simulink model "biomasav_2"  (R2018a)
settings: Solver=ode8  StartTime=0.0  StopTime=10.0  FixedStep=0.0001  RelTol=1e-3
InitFcn:
  | SimulinkInit_linea_transmision
values from neighbouring files (symbols this model uses):
  b = 4.91    [SimulinkInit_linea_transmision.m]
  C = 1    [SimulinkInit_linea_transmision.m]
  C1 = 22e-6    (= 2.2e-05)    [SimulinkInit_linea_transmision.m]
  C2 = 22e-6    (= 2.2e-05)    [SimulinkInit_linea_transmision.m]
  C3 = 610e-6    (= 0.00061)    [SimulinkInit_linea_transmision.m]
  Cl = 20000e-6    (= 0.02)    [SimulinkInit_linea_transmision.m]
  Jd = 0.3    [SimulinkInit_linea_transmision.m]
  K = 25    [SimulinkInit_linea_transmision.m]    (also in uio_linear.m = K1+E*H)
  K1 = 9.66    [SimulinkInit_linea_transmision.m]    (also in uio_linear.m = K1')
  K11 = 0.8    [SimulinkInit_linea_transmision.m]
  K1d = 1.15    [SimulinkInit_linea_transmision.m]
  K2 = 6.97    [SimulinkInit_linea_transmision.m]
  K22 = 0.2    [SimulinkInit_linea_transmision.m]
  K2d = 1    [SimulinkInit_linea_transmision.m]
  K3 = 31.8    [SimulinkInit_linea_transmision.m]
  K33 = 0.23    [SimulinkInit_linea_transmision.m]
  K3d = 1    [SimulinkInit_linea_transmision.m]
  K4 = 15.1    [SimulinkInit_linea_transmision.m]
  Kd = 0.02    [SimulinkInit_linea_transmision.m]
  Kdc = 0.02    [SimulinkInit_linea_transmision.m]
  Kf = 1    [SimulinkInit_linea_transmision.m]
  Kh = 1.2    [SimulinkInit_linea_transmision.m]
  Ks = 21.5    [SimulinkInit_linea_transmision.m]
  Ksc = 3    [SimulinkInit_linea_transmision.m]
  Kv = 1    [SimulinkInit_linea_transmision.m]
  L = 5.2    [SimulinkInit_linea_transmision.m]
  L1 = 40e-3    (= 0.04)    [SimulinkInit_linea_transmision.m]
  L2 = 30e-3    (= 0.03)    [SimulinkInit_linea_transmision.m]
  L3 = 5e-3    (= 0.005)    [SimulinkInit_linea_transmision.m]
  L4 = 35e-6    (= 3.5e-05)    [SimulinkInit_linea_transmision.m]
  L5 = 22e-6    (= 2.2e-05)    [SimulinkInit_linea_transmision.m]
  L6 = 10e-6    (= 1e-05)    [SimulinkInit_linea_transmision.m]
  Pd = 0.1    [SimulinkInit_linea_transmision.m]
  R = 10    [SimulinkInit_linea_transmision.m]
  R1 = 0.1    [SimulinkInit_linea_transmision.m]
  R2 = 0.2    [SimulinkInit_linea_transmision.m]
  R3 = 1e-3    (= 0.001)    [SimulinkInit_linea_transmision.m]
  R4 = 0.005    [SimulinkInit_linea_transmision.m]
  R5 = 0.0012    [SimulinkInit_linea_transmision.m]
  R6 = 0.001    [SimulinkInit_linea_transmision.m]
  RL = 10    [SimulinkInit_linea_transmision.m]
  Sbin = 13.8    [SimulinkInit_linea_transmision.m]
  Svin = 2.91    [SimulinkInit_linea_transmision.m]
  T1 = 0.4    [SimulinkInit_linea_transmision.m]
  T2 = 1    [SimulinkInit_linea_transmision.m]
  T3 = 15    [SimulinkInit_linea_transmision.m]
  T4 = 2.5    [SimulinkInit_linea_transmision.m]
  T5 = 3.3    [SimulinkInit_linea_transmision.m]
  Tao1d = 0.5    [SimulinkInit_linea_transmision.m]
  Tao2d = 0.125    [SimulinkInit_linea_transmision.m]
  Tcd = 0.2    [SimulinkInit_linea_transmision.m]
  Tcr = 0.01    [SimulinkInit_linea_transmision.m]
  Tf = 0.04    [SimulinkInit_linea_transmision.m]
  Tr = 950    [SimulinkInit_linea_transmision.m]
  Tt = 450    [SimulinkInit_linea_transmision.m]
  Ttd = 0.04    [SimulinkInit_linea_transmision.m]
  Tv = 0.05    [SimulinkInit_linea_transmision.m]
  V = 20    [SimulinkInit_linea_transmision.m]
  wref = 70000    [SimulinkInit_linea_transmision.m]
  X_acid = 1.2    [SimulinkInit_linea_transmision.m]
  X_meth = 0.35    [SimulinkInit_linea_transmision.m]
  Z = 3    [SimulinkInit_linea_transmision.m]
libraries: dsparch4 x4, powerlib_meascontrol x2, simulink x1
settings Model: Creator=MarioAndres  LastModifiedBy=cmparedes
settings OptimizationCC: DefaultParameterBehavior=Inlined  EnhancedBackFolding=on  PassReuseOutputArgsAs=Individual arguments  OptimizeBlockOrder=speed  DifferentSizesBufferReuse=on  OptimizationCustomize=off
settings DebuggingCC: ParameterTunabilityLossMsg=error
settings HardwareCC: TargetBitPerPointer=64  TargetBitPerSizeT=64  TargetBitPerPtrDiffT=64  TargetLongLongMode=on  TargetIntDivRoundTo=Zero  TargetEndianess=LittleEndian  TargetWordSize=64  TargetHWDeviceType=MATLAB Host  ProdEqTarget=off
settings SFSimCC: MATLABDynamicMemAlloc=off
settings RTWCC: SystemTargetFile=ert.tlc  TemplateMakefile=ert_default_tmf  GenerateReport=on  IncludeHyperlinkInReport=on  LaunchReport=on  GenerateTraceInfo=on  GenerateTraceReport=on  GenerateTraceReportSl=on  GenerateTraceReportSf=on  GenerateTraceReportEml=on
settings CodeAppCC: ForceParamTrailComments=on  IgnoreCustomStorageClasses=off  OperatorAnnotations=on  SimulinkDataObjDesc=on  SFDataObjDesc=on  InsertBlockDesc=on
settings ERTTargetCC: TargetLangStandard=C99 (ISO)  GenerateSampleERTMain=on  SupportContinuousTime=on  InlinedParameterPlacement=NonHierarchical  ERTCustomFileTemplate=example_file_process.tlc

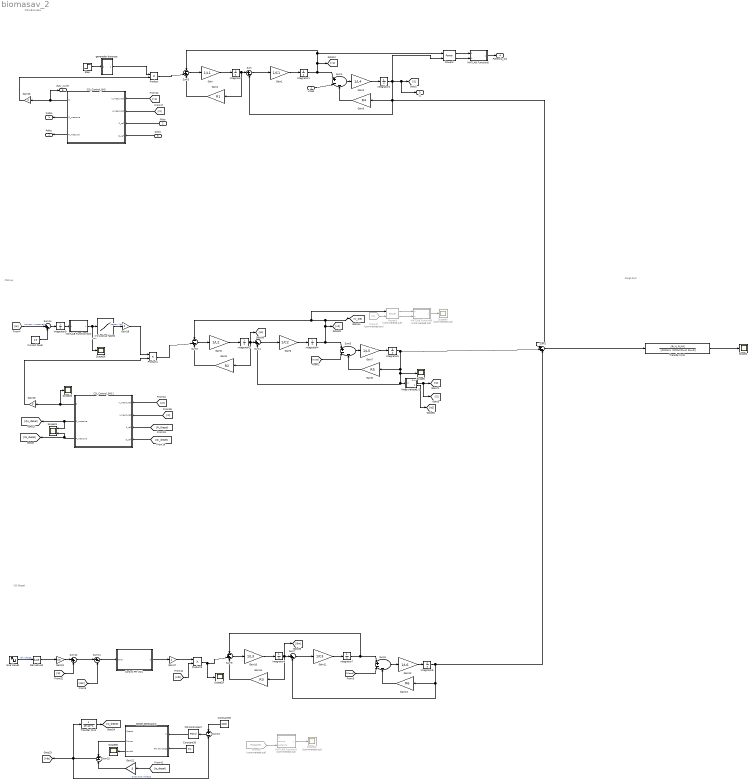
== system biomasav_2 ==
  note: CSI1-Biomasa
  note: CSI2-pv
  note: VSI-Diesel
  note: Carga RLC
  Vload : Inport
  Pibio : Inport  Port=2
  Qibio : Inport  Port=3
  1-D Lookup Table2 : Lookup_n-D  NumberOfTableDimensions=1  BreakpointsForDimension1=[0 10 20 30 40 50 70 80 100]  Table=[0 10 200 500 800 1000 1140 1150 1200]  InternalRulePriority=Speed  RndMeth=Simplest  InputSameDT=on
  CSI_Control_BIO : Subsystem  mask{A=[0.0201   -0.039932     0.01986], B=[1     -1.9966       0.998], T=0.0001, st_time=.1, Dn=[1     -1.0364], Dd=[1    -0.96364]}
      mask prompts: A "Numerador del control PR(z)"; B "Denominador del control PR(z)"; T "Tiempo de muestreo"; st_time "Tiempo_muerto"; Dn "Dn (Numerador de D(z))"; Dd "Dd (numerador de D(z))"
      mask DialogControl descripcion Prompt: Lazo de control de corriente para inversor monofasico. La entrada es un setpoint de potencia [P, Q]. Con ese setpoint se calcula la referencia de corriente sinusoidal deacuerdo a la tension medida de la red. Por lo anterior este controlador solo es valido para un inversor conectado a la red pues hara que se comporte como un CSI.
      mask DialogControl Control2 Prompt: Dn y Dd corresponden al numerador y denominador de la funcion de transferencia en Z (denominada D(z)) que hara un desfase de 90 de las señales medidas de tension y corriente del inversor. Estos desfases permiten mimificar las señales alfa y beta, de esta forma usar la misma teoria de potencia instantanea para el caso monofasico.
  CSI_Control_BIO1 : Subsystem  mask{A=[0.0201   -0.039932     0.01986], B=[1     -1.9966       0.998], T=0.0001, st_time=0, Dn=[1     -1.0364], Dd=[1    -0.96364]}
      mask prompts: A "Numerador del control PR(z)"; B "Denominador del control PR(z)"; T "Tiempo de muestreo"; st_time "Tiempo_muerto"; Dn "Dn (Numerador de D(z))"; Dd "Dd (numerador de D(z))"
      mask DialogControl descripcion Prompt: Lazo de control de corriente para inversor monofasico. La entrada es un setpoint de potencia [P, Q]. Con ese setpoint se calcula la referencia de corriente sinusoidal deacuerdo a la tension medida de la red. Por lo anterior este controlador solo es valido para un inversor conectado a la red pues hara que se comporte como un CSI.
      mask DialogControl Control2 Prompt: Dn y Dd corresponden al numerador y denominador de la funcion de transferencia en Z (denominada D(z)) que hara un desfase de 90 de las señales medidas de tension y corriente del inversor. Estos desfases permiten mimificar las señales alfa y beta, de esta forma usar la misma teoria de potencia instantanea para el caso monofasico.
  Constant29 : Constant  Value=1000
  Constant30 : Constant  Value=0.1
  Control PR VSI1 : Subsystem
  Current Panel : Constant  Value=1.5
  Derivative2 : Derivative  CoefficientInTFapproximation=0
  Diesel Generator2 : Subsystem
  From37 : From  Commented=on  GotoTag=Papadiel
  From47 : From  Commented=on  GotoTag=i2
  Gain : Gain  Gain=1/L1
  Gain1 : Gain  Gain=1/C1
  Gain10 : Gain  Gain=1/L3
  Gain11 : Gain  Gain=1/C3
  Gain12 : Gain  Gain=1/L6
  Gain13 : Gain  Gain=R6
  Gain14 : Gain  Gain=R3
  Gain{15..18} (4 alike) : Gain  Gain=2
  Gain19 : Gain  Gain=C3
  Gain2 : Gain  Gain=1/L4
  Gain21 : Gain  Gain=.5
  Gain3 : Gain  Gain=R4
  Gain4 : Gain  Gain=R1
  Gain5 : Gain  Gain=1/L2
  Gain6 : Gain  Gain=1/C2
  Gain7 : Gain  Gain=1/L5
  Gain8 : Gain  Gain=R5
  Gain9 : Gain  Gain=R2
  Integrator{,1..8} (9 alike) : Integrator
  Integrator9 : Integrator  LimitOutput=on  UpperSaturationLimit=1  LowerSaturationLimit=0
  "MATLAB Function SOC " : MATLAB Function  TreatAsAtomicUnit=on
  MATLAB Function3 : MATLAB Function  Commented=on  TreatAsAtomicUnit=on
  MATLAB Function5 : MATLAB Function  TreatAsAtomicUnit=on
  MATLAB Function6 : MATLAB Function  Commented=on  TreatAsAtomicUnit=on
  MeasureNode_I1 : Subsystem
  PID Controller2 : simulink/Continuous/PID Controller  Controller=PID  TimeDomain=Continuous-time  SampleTime=-1  IntegratorMethod=Forward Euler  FilterMethod=Forward Euler  Form=Parallel  UseFilter=on  ControllerParametersSource=internal  P=0.000853612192208084  I=3.94394231511782e-05  D=0.00224356290205903  N=0.155980576752107  InitialConditionSource=internal  InitialConditionForIntegrator=0  InitialConditionForFilter=0  ExternalReset=none  LimitOutput=off  UpperSaturationLimit=inf  LowerSaturationLimit=-inf  LinearizeAsGain=on  AntiWindupMode=none  Kb=1  TrackingMode=off  Kt=1  PParamMin=[]  PParamMax=[]  IParamMin=[]  IParamMax=[]  DParamMin=[]  DParamMax=[]  NParamMin=[]  NParamMax=[]  KbParamMin=[]  KbParamMax=[]  KtParamMin=[]  KtParamMax=[]  POutMin=[]  POutMax=[]  IOutMin=[]  IOutMax=[]  DOutMin=[]  DOutMax=[]  NOutMin=[]  NOutMax=[]  KbOutMin=[]  KbOutMax=[]  KtOutMin=[]  KtOutMax=[]  IntegratorOutMin=[]  IntegratorOutMax=[]  FilterOutMin=[]  FilterOutMax=[]  SumOutMin=[]  SumOutMax=[]  SumI1OutMin=[]  SumI1OutMax=[]  SumI2OutMin=[]  SumI2OutMax=[]  SumI3OutMin=[]  SumI3OutMax=[]  SumDOutMin=[]  SumDOutMax=[]  SaturationOutMin=[]  SaturationOutMax=[]  IntegratorContinuousStateAttributes=''  IntegratorStateMustResolveToSignalObject=off  IntegratorRTWStateStorageClass=Auto  FilterContinuousStateAttributes=''  FilterStateMustResolveToSignalObject=off  FilterRTWStateStorageClass=Auto  DifferentiatorICPrevScaledInput=0  DifferentiatorOutMin=[]  DifferentiatorOutMax=[]  InitialConditionSetting=State (most efficient)  FilterDiffOutCoefMin=[]  FilterDiffOutCoefMax=[]  SumDenOutMin=[]  SumDenOutMax=[]  SumNumOutMin=[]  SumNumOutMax=[]  ReciprocalOutMin=[]  ReciprocalOutMax=[]  DivideOutMin=[]  DivideOutMax=[]  TunerSelectOption=Transfer Function Based (PID Tuner App)
  Power3 : powerlib_meascontrol/Measurements/Power  Freq=60  Vinit=[1, 0]  Iinit=[1, 0]  Ts=0
      settings: SourceProductName=Simscape Power Systems
  Power4 : powerlib_meascontrol/Measurements/Power  Commented=on  Freq=60  Vinit=[1, 0]  Iinit=[1, 0]  Ts=0
      settings: SourceProductName=Simscape Power Systems
  Product : Product
  Product1 : Product
  Product3 : Product
  Scope{2,5,20,26,29,38} (6 alike) : Scope
  Scope21 : Scope  NumInputPorts=2
  Scope22 : Scope  Commented=on
  Scope40 : Scope  Commented=on
  Sine Wave1 : Sin  Amplitude=170  Frequency=2*pi*60  SampleTime=0
  Step : Step  Time=0  After=28  SampleTime=0
  Sum{,4,7,11} (4 alike) : Sum  Inputs=|+-
  Sum1 : Sum  Inputs=|+--
  Sum12 : Sum  Inputs=|++
  Sum13 : Sum  Inputs=+-
  Sum14 : Sum  Inputs=|++
  Sum15 : Sum  Inputs=+-
  Sum2 : Sum  Inputs=|+++
  Sum3 : Sum  Inputs=-|+-
  Sum5 : Sum  Inputs=|+--
  Sum6 : Sum  Inputs=-|+-
  Sum8 : Sum  Inputs=|+--
  Sum9 : Sum  Inputs=-|+-
  Transfer Fcn3 : TransferFcn  Numerator=[RL*L RL*R]  Denominator="[Cl*RL*L  (R*RL*Cl+L) RL+R]"
  Transfer Fcn4 : TransferFcn  Denominator=[1e-4 1]
  generador biomasa : Subsystem
  Qobio : Outport
  Pobio : Outport  Port=2
  i1 : Outport  Port=3
  Potencia_bio : Outport  Port=4
  duty_cycle : Outport  Port=5
  wires:
  MATLAB Function5/1(y) -> Potencia_bio/1
  CSI_Control_BIO/1(D) -> duty_cycle/1, Gain15/1
  Product/1 -> Sum3/2
  [i1] -> CSI_Control_BIO/2(I_measured)
  generador biomasa/1(Vdc) -> Product/1
  Step/1 -> generador biomasa/1(In1)
  Gain15/1 -> Product/2
  [v1] -> CSI_Control_BIO/1(V_measured)
  Sum/1 -> Gain1/1
  Sum3/1 -> Gain/1
  Gain4/1 -> Sum3/3
  Integrator1/1 -> [v1], Sum3/1, Power3/1, Sum1/1
  Gain2/1 -> Integrator2/1
  Sum1/1 -> Gain2/1
  Power3/1 -> MATLAB Function5/1(p)
  Gain1/1 -> Integrator1/1
  Power3/2 -> MATLAB Function5/2(q)
  Integrator/1 -> Gain4/1, Sum/1
  Gain/1 -> Integrator/1
  Gain3/1 -> Sum1/3
  Pibio/1 -> CSI_Control_BIO/3(P_ref)
  Qibio/1 -> CSI_Control_BIO/4(Q_ref)
  Vload/1 -> Sum1/2
  CSI_Control_BIO/2(Q_measure) -> Qobio/1
  CSI_Control_BIO/3(P_measure) -> Pobio/1
  [i2] -> CSI_Control_BIO1/2(I_measured)
  [Qi_diesel] -> CSI_Control_BIO1/4(Q_ref)
  Gain16/1 -> Product1/2
  Sum6/1 -> Gain5/1
  [i3] -> Sum12/2
  Gain11/1 -> Integrator7/1
  MeasureNode_I1/2(Out1) -> [a2]
  MATLAB Function3/1(y) -> Scope22/1
  Current Panel/1 -> Sum14/2
  MATLAB Function6/1(y) -> Scope40/1
  Gain17/1 -> Product3/1
  CSI_Control_BIO1/1(D) -> Scope20/1, Gain16/1
  Sum8/1 -> Gain12/1
  PID Controller2/1 -> Diesel Generator2/1(in)
  [i3m] -> Sum11/2
  Sum15/1 -> [Vdc], Sum13/2, Transfer Fcn4/1  "Output DC Voltage"
  [Vload] -> Sum8/2
  "MATLAB Function SOC "/1(y) -> Scope26/1, 1-D Lookup Table2/1  "soc"
  Diesel Generator2/2(Power) -> Sum15/1
  Sum9/1 -> Gain10/1
  Gain5/1 -> Integrator3/1
  [v2] -> CSI_Control_BIO1/1(V_measured)
  Gain6/1 -> Integrator4/1
  Power4/1 -> MATLAB Function6/1(p)
  [Pi_Diesel] -> CSI_Control_BIO1/3(P_ref)
  Power4/2 -> MATLAB Function6/2(q)
  Constant29/1 -> Sum13/1
  Gain21/1 -> Sum15/2
  [Vdc] -> Product3/2
  Diesel Generator2/3(caudal) -> Scope38/1
  Transfer Fcn4/1 -> [Io_diesel]
  Constant30/1 -> Diesel Generator2/2(Par de Carga)
  From37/1 -> MATLAB Function3/3(potencia)
  Sum13/1 -> PID Controller2/1
  Integrator4/1 -> [v2], [V_die], Power4/1, Sum6/1, Sum5/1
  Sum14/1 -> Integrator9/1
  Gain18/1 -> Product1/1
  Sum11/1 -> Control PR VSI1/1(Ierror)
  Gain13/1 -> Sum8/3
  Derivative2/1 -> Gain19/1
  1-D Lookup Table2/1 -> Gain18/1  "battery Vdc"
  Integrator9/1 -> "MATLAB Function SOC "/1(u)
  Product1/1 -> Sum6/2
  From47/1 -> Power4/2
  Sum4/1 -> Gain6/1
  Control PR VSI1/1(d) -> Gain17/1
  Product3/1 -> Sum9/2, Scope29/1
  Integrator7/1 -> Sum9/1, Sum8/1
  Integrator5/1 -> Sum2/2, Scope5/1, MeasureNode_I1/1(in), Sum4/2, Gain8/1
  Gain7/1 -> Integrator5/1
  [Io_diesel] -> Gain21/1
  [Vload] -> Sum5/2
  CSI_Control_BIO1/3(P_measure) -> [Po_diesel], Scope21/2
  Gain12/1 -> Integrator8/1
  CSI_Control_BIO1/2(Q_measure) -> [Qo_diesel], Scope21/1
  Transfer Fcn3/1 -> Scope2/1
  Gain8/1 -> Sum5/3
  Sine Wave1/1 -> Derivative2/1  "ref voltage"
  Gain9/1 -> Sum6/3
  [ipi] -> Sum14/1  "inductor I measured"
  Gain10/1 -> Integrator6/1
  Integrator2/1 -> Power3/2, Sum2/1, Sum/2, Gain3/1, i1/1, [i1]
  Gain19/1 -> Sum12/1
  Sum5/1 -> Gain7/1
  Gain14/1 -> Sum9/3
  Sum2/1 -> Transfer Fcn3/1
  Integrator8/1 -> Sum2/3, Gain13/1, Sum7/2
  Sum12/1 -> Sum11/1
  Integrator6/1 -> [i3m], Gain14/1, Sum7/1
  MeasureNode_I1/1(Out) -> [i2], [I2]
  Integrator3/1 -> [ipi], Gain9/1, Sum4/1
  Sum7/1 -> Gain11/1

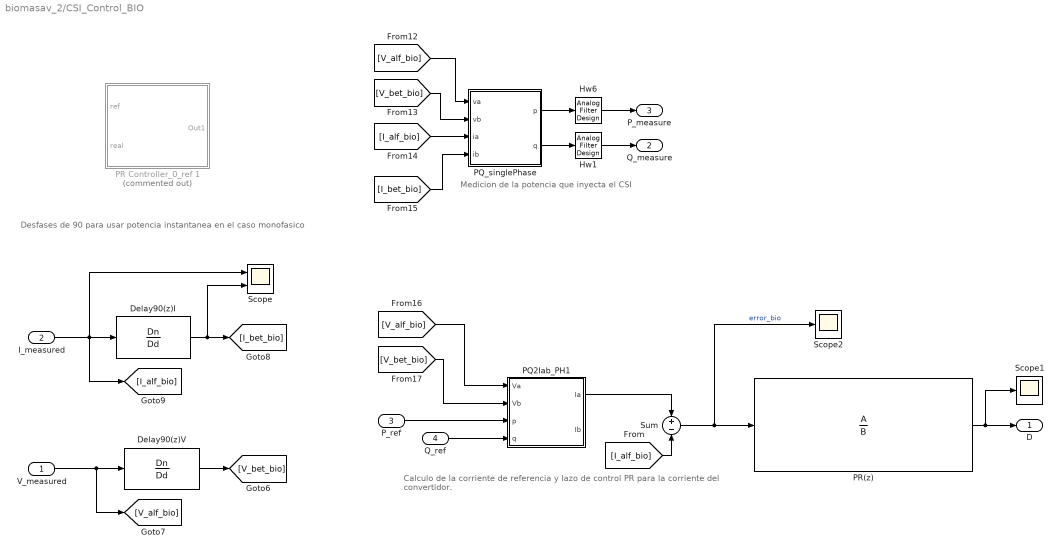
== system biomasav_2/CSI_Control_BIO ==
  note: Medicion de la potencia que inyecta el CSI
  note: Desfases de 90 para usar potencia
      | instantanea en el caso monofasico
  note: Calculo de la corriente de referencia
      | y lazo de control PR para la corriente
      | del convertidor.
  V_measured : Inport
  I_measured : Inport  Port=2
  P_ref : Inport  Port=3
  Q_ref : Inport  Port=4
  Delay90(z)I : DiscreteTransferFcn  Numerator=Dn  Denominator=Dd  SampleTime=T
  Delay90(z)V : DiscreteTransferFcn  Numerator=Dn  Denominator=Dd  SampleTime=T
  Hw1 : dsparch4/Analog Filter Design  method=Bessel  filttype=Lowpass  N=4  Wlo=30*2*pi  Whi=80  Rp=2  Rs=80
  Hw6 : dsparch4/Analog Filter Design  method=Bessel  filttype=Lowpass  N=4  Wlo=30*2*pi  Whi=80  Rp=2  Rs=80
  PQ2Iab_PH1 : MATLAB Function  TreatAsAtomicUnit=on
  PQ_singlePhase : MATLAB Function  TreatAsAtomicUnit=on
  PR Controller_0_ref 1 : Subsystem  Commented=on  mask{Kp=40/100, Ki=200, wa=2, w0=60*2*pi, st_time=1e-3}
      mask prompts: Kp "Ganancia Proporcional"; Ki "Ganancia Integral"; wa "Ancho camapana resonancia"; w0 "Frecuencia Central"; st_time "Tiempo muerto (Start)"
      mask Display:
      | port_label('input',1,'ref')
      | port_label('input',2,'sens')
      | port_label('output',1,'out')
      | 
      | plot(.4+[0:.01:pi/10], .32+sin(40*[0:.01:pi/10])/13)
      | 
      | plot([.4 .6],.05+[.5 .7])
      | plot([.4 .6],.05+[.9 .7])
      | plot([.4 .4],.05+[.9 .5])
      | 
      | text(.27,.37,'\fontsize{25} \int', 'texmode', 'on')
  PR(z) : DiscreteTransferFcn  Numerator=A  Denominator=B  SampleTime=T
  Scope : Scope  NumInputPorts=2
  Scope1 : Scope
  Scope2 : Scope
  Sum : Sum  Inputs=+-
  D : Outport
  Q_measure : Outport  Port=2
  P_measure : Outport  Port=3
  wires:
  I_measured/1 -> Scope/1, Delay90(z)I/1, [I_alf_bio]
  [V_bet_bio] -> PQ2Iab_PH1/2(Vb)
  Delay90(z)I/1 -> Scope/2, [I_bet_bio]
  [I_bet_bio] -> PQ_singlePhase/4(ib)
  [I_alf_bio] -> PQ_singlePhase/3(ia)
  [V_alf_bio] -> PQ2Iab_PH1/1(Va)
  Delay90(z)V/1 -> [V_bet_bio]
  [V_bet_bio] -> PQ_singlePhase/2(vb)
  [V_alf_bio] -> PQ_singlePhase/1(va)
  V_measured/1 -> Delay90(z)V/1, [V_alf_bio]
  P_ref/1 -> PQ2Iab_PH1/3(p)
  Q_ref/1 -> PQ2Iab_PH1/4(q)
  Sum/1 -> Scope2/1, PR(z)/1  "error_bio"
  [I_alf_bio] -> Sum/2
  PQ2Iab_PH1/1(Ia) -> Sum/1
  PR(z)/1 -> Scope1/1, D/1
  PQ_singlePhase/2(q) -> Hw1/1
  Hw1/1 -> Q_measure/1
  PQ_singlePhase/1(p) -> Hw6/1
  Hw6/1 -> P_measure/1

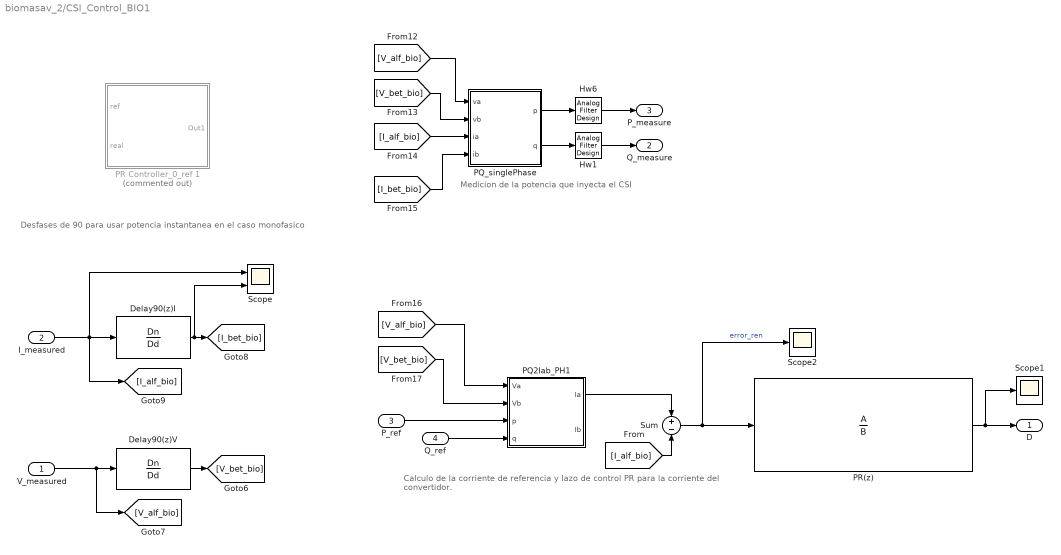
== system biomasav_2/CSI_Control_BIO1 ==
  note: Medicion de la potencia que inyecta el CSI
  note: Desfases de 90 para usar potencia
      | instantanea en el caso monofasico
  note: Calculo de la corriente de referencia
      | y lazo de control PR para la corriente
      | del convertidor.
  V_measured : Inport
  I_measured : Inport  Port=2
  P_ref : Inport  Port=3
  Q_ref : Inport  Port=4
  Delay90(z)I : DiscreteTransferFcn  Numerator=Dn  Denominator=Dd  SampleTime=T
  Delay90(z)V : DiscreteTransferFcn  Numerator=Dn  Denominator=Dd  SampleTime=T
  Hw1 : dsparch4/Analog Filter Design  method=Bessel  filttype=Lowpass  N=4  Wlo=30*2*pi  Whi=80  Rp=2  Rs=80
  Hw6 : dsparch4/Analog Filter Design  method=Bessel  filttype=Lowpass  N=4  Wlo=30*2*pi  Whi=80  Rp=2  Rs=80
  PQ2Iab_PH1 : MATLAB Function  TreatAsAtomicUnit=on
  PQ_singlePhase : MATLAB Function  TreatAsAtomicUnit=on
  PR Controller_0_ref 1 : Subsystem  Commented=on  mask{Kp=40/100, Ki=200, wa=2, w0=60*2*pi, st_time=1e-3}
      mask prompts: Kp "Ganancia Proporcional"; Ki "Ganancia Integral"; wa "Ancho camapana resonancia"; w0 "Frecuencia Central"; st_time "Tiempo muerto (Start)"
      mask Display:
      | port_label('input',1,'ref')
      | port_label('input',2,'sens')
      | port_label('output',1,'out')
      | 
      | plot(.4+[0:.01:pi/10], .32+sin(40*[0:.01:pi/10])/13)
      | 
      | plot([.4 .6],.05+[.5 .7])
      | plot([.4 .6],.05+[.9 .7])
      | plot([.4 .4],.05+[.9 .5])
      | 
      | text(.27,.37,'\fontsize{25} \int', 'texmode', 'on')
  PR(z) : DiscreteTransferFcn  Numerator=A  Denominator=B  SampleTime=T
  Scope : Scope  NumInputPorts=2
  Scope1 : Scope
  Scope2 : Scope
  Sum : Sum  Inputs=+-
  D : Outport
  Q_measure : Outport  Port=2
  P_measure : Outport  Port=3
  wires:
  I_measured/1 -> Scope/1, Delay90(z)I/1, [I_alf_bio]
  [V_bet_bio] -> PQ2Iab_PH1/2(Vb)
  Delay90(z)I/1 -> Scope/2, [I_bet_bio]
  [I_bet_bio] -> PQ_singlePhase/4(ib)
  [I_alf_bio] -> PQ_singlePhase/3(ia)
  [V_alf_bio] -> PQ2Iab_PH1/1(Va)
  Delay90(z)V/1 -> [V_bet_bio]
  [V_bet_bio] -> PQ_singlePhase/2(vb)
  [V_alf_bio] -> PQ_singlePhase/1(va)
  V_measured/1 -> Delay90(z)V/1, [V_alf_bio]
  P_ref/1 -> PQ2Iab_PH1/3(p)
  Q_ref/1 -> PQ2Iab_PH1/4(q)
  Sum/1 -> Scope2/1, PR(z)/1  "error_ren"
  [I_alf_bio] -> Sum/2
  PQ2Iab_PH1/1(Ia) -> Sum/1
  PR(z)/1 -> Scope1/1, D/1
  PQ_singlePhase/2(q) -> Hw1/1
  Hw1/1 -> Q_measure/1
  PQ_singlePhase/1(p) -> Hw6/1
  Hw6/1 -> P_measure/1

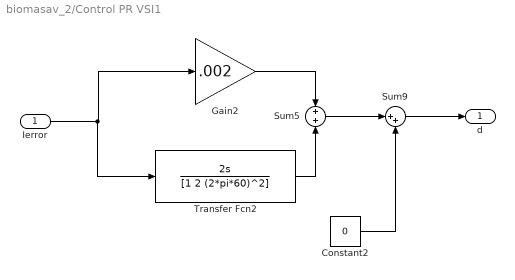
== system biomasav_2/Control PR VSI1 ==
  Ierror : Inport
  Constant2 : Constant  Value=0
  Gain2 : Gain  Gain=.002
  Sum5 : Sum  Inputs=+|+
  Sum9 : Sum  Inputs=|++
  Transfer Fcn2 : TransferFcn  Numerator=[2 0]  Denominator=[1 2 (2*pi*60)^2]
  d : Outport
  wires:
  Constant2/1 -> Sum9/2
  Sum5/1 -> Sum9/1
  Transfer Fcn2/1 -> Sum5/2
  Gain2/1 -> Sum5/1
  Ierror/1 -> Transfer Fcn2/1, Gain2/1
  Sum9/1 -> d/1

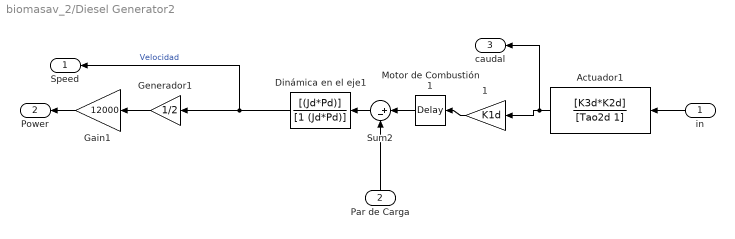
== system biomasav_2/Diesel Generator2 ==
  in : Inport
  Par de Carga : Inport  Port=2
  " 1" : Gain  Gain=K1d
  " Generador1" : Gain  Gain=1/2
  Actuador1 : TransferFcn  Numerator=[K3d*K2d]  Denominator=[Tao2d 1]
  Dinámica en el eje1 : TransferFcn  Numerator=[(Jd*Pd)]  Denominator=[1 (Jd*Pd)]
  Gain1 : Gain  Gain=12000
  Motor de Combustión1 : TransportDelay  DelayTime=Tao1d
  Sum2 : Sum  Inputs=|+-
  Speed : Outport
  Power : Outport  Port=2
  caudal : Outport  Port=3
  wires:
  " 1"/1 -> Motor de Combustión1/1
  " Generador1"/1 -> Gain1/1
  Motor de Combustión1/1 -> Sum2/1
  Actuador1/1 -> caudal/1, " 1"/1
  Dinámica en el eje1/1 -> Speed/1, " Generador1"/1  "Velocidad"
  Sum2/1 -> Dinámica en el eje1/1
  in/1 -> Actuador1/1
  Par de Carga/1 -> Sum2/2
  Gain1/1 -> Power/1

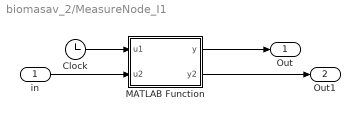
== system biomasav_2/MeasureNode_I1 ==
  in : Inport
  Clock : Clock
  MATLAB Function : MATLAB Function  TreatAsAtomicUnit=on
  Out : Outport
  Out1 : Outport  Port=2
  wires:
  MATLAB Function/1(y) -> Out/1
  Clock/1 -> MATLAB Function/1(u1)
  in/1 -> MATLAB Function/2(u2)
  MATLAB Function/2(y2) -> Out1/1

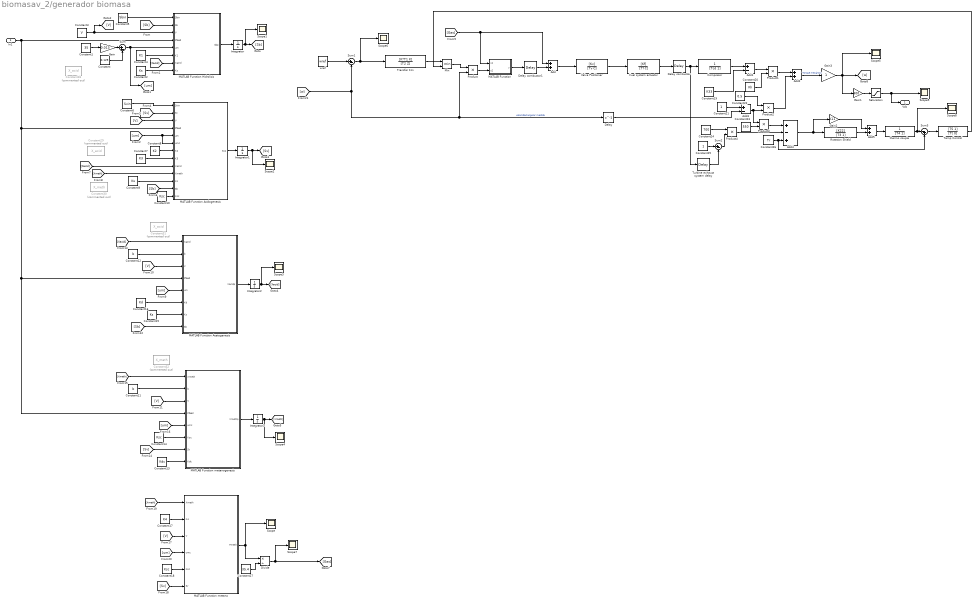
== system biomasav_2/generador biomasa ==
  In1 : Inport
  Add : Sum
  Add1 : Sum  Inputs=+-
  Add2 : Sum
  Add3 : Sum  Inputs=+-
  Add4 : Sum  Inputs=+-+
  Add5 : Sum
  Compresor : TransferFcn  Denominator=[Tcd 1]
  Constant : Constant  Value=0.129
  Constant1 : Constant  Value=35
  Constant10 : Constant  Value=Ksc
  Constant11 : Constant  Value=b
  Constant12 : Constant  Value=b
  Constant13 : Constant  Value=Kdc
  Constant14 : Constant  Value=Ksc
  Constant15 : Constant  Value=Ks
  Constant16 : Constant  Value=Kd
  Constant17 : Constant  Value=K4
  Constant18 : Constant  Value=Ksc
  Constant19 : Constant  Value=K33
  Constant2 : Constant  Value=Ks
  Constant20 : Constant  Value=Kh
  Constant21 : Constant
  Constant22 : Constant  Value=0.5
  Constant23 : Constant  Value=550
  Constant24 : Constant  Value=700
  Constant25 : Constant
  Constant26 : Constant  Value=Tr
  Constant27 : Constant  Value=35.4
  Constant28 : Constant  Commented=on  Value=X_acid
  Constant29 : Constant  Commented=on  Value=X_acid
  Constant3 : Constant  Value=V
  Constant30 : Constant  Commented=on  Value=X_meth
  Constant31 : Constant  Commented=on  Value=X_acid
  Constant32 : Constant  Commented=on  Value=X_meth
  Constant4 : Constant  Value=K1
  Constant5 : Constant  Value=Sbin
  Constant6 : Constant  Value=Svin
  Constant7 : Constant  Value=K3
  Constant8 : Constant  Value=K2
  Constant9 : Constant  Value=Ks
  Delay : Delay  DelayLength=1
  Delay combustor : TransportDelay  DelayTime=Tcr
  Delay combustor1 : TransportDelay  DelayTime=0
  Divide : Product  Inputs=*/
  Fuel system actuator : TransferFcn  Numerator=[Kf]  Denominator=[Tf C]
  Gain : Gain  Gain=0.013
  Gain1 : Gain  Gain=900
  Gain2 : Gain  Gain=K11
  Gain3 : Gain
  Integrator : Integrator
  Integrator1 : Integrator
  Integrator2 : Integrator  InitialCondition=1.2
  Integrator3 : Integrator  InitialCondition=0.35
  MATLAB Function : MATLAB Function  TreatAsAtomicUnit=on
  MATLAB Function Acetogenesis : MATLAB Function  TreatAsAtomicUnit=on
  MATLAB Function Acidogenesis : MATLAB Function  TreatAsAtomicUnit=on
  MATLAB Function Hidrolisis : MATLAB Function  TreatAsAtomicUnit=on
  MATLAB Function metano : MATLAB Function  TreatAsAtomicUnit=on
  MATLAB Function metanogenesis : MATLAB Function  TreatAsAtomicUnit=on
  Min : MinMax  Inputs=2
  Product{,1..4} (5 alike) : Product
  Rotation Shield : TransferFcn  Numerator=[K22]  Denominator=[T3 1]
  Saturation : Saturate  UpperLimit=1000  LowerLimit=0
  Scope{,1..9} (10 alike) : Scope
  Sum : Sum  Inputs=|+-
  Sum1 : Sum  Inputs=|+-
  Sum2 : Sum  Inputs=|+-
  Sum3 : Sum  Inputs=|-+
  Temp Control : TransferFcn  Numerator=[T5 1]  Denominator=[Tt 0]
  Transfer Fcn : TransferFcn  Numerator=[K*T1 K]  Denominator=[T2 Z]
  Turbine exhaust system delay : TransportDelay  DelayTime=Ttd
  Valve Positioner : TransferFcn  Numerator=[Kv]  Denominator=[Tv C]
  thermo couple : TransferFcn  Denominator=[T4 1]
  wref : Constant  Value=wref
  Vdc : Outport
  wires:
  MATLAB Function metano/1(Fmeth) -> Divide/1, Scope/1
  Sum/1 -> [um], MATLAB Function Hidrolisis/5(um)
  Constant16/1 -> MATLAB Function Acetogenesis/6(Kd)
  Temp Control/1 -> Min/2
  Integrator/1 -> Scope1/1, [Sb]
  Gain3/1 -> Gain1/1, Scope5/1, [w]
  Sum1/1 -> Transfer Fcn/1, Scope6/1
  [Sb] -> MATLAB Function Acetogenesis/8(Sb)
  [Sv] -> MATLAB Function metanogenesis/7(Sv)
  Add4/1 -> Rotation Shield/1, Gain2/1
  Constant8/1 -> MATLAB Function Acidogenesis/7(K2)
  Constant24/1 -> Product4/1
  [V] -> MATLAB Function Acetogenesis/3(V)
  Constant23/1 -> Product3/2
  Constant27/1 -> Divide/2
  [Sb] -> MATLAB Function Acidogenesis/12(Sb)
  Integrator3/1 -> Scope4/1, [Xmeth]
  Integrator2/1 -> Scope3/1, [Xacid]
  Divide/1 -> Scope7/1, [Gas]
  Constant7/1 -> MATLAB Function Acidogenesis/8(K3)
  Delay combustor/1 -> Turbine exhaust system delay/1, Compresor/1
  [V] -> MATLAB Function Acidogenesis/3(V)
  Constant12/1 -> MATLAB Function Acetogenesis/2(b)
  Sum2/1 -> Product4/2
  [V] -> MATLAB Function metanogenesis/3(V)
  Gain/1 -> Sum/1
  Product/1 -> MATLAB Function/2(u2)
  [w] -> Product/2, Delay/1, Sum1/2  "velocidad angular medida"
  Constant6/1 -> MATLAB Function Acidogenesis/1(Svin)
  wref/1 -> Sum1/1
  [Gas] -> MATLAB Function/1(u1), Add/1
  [Sv] -> MATLAB Function metano/6(Sv)
  MATLAB Function Hidrolisis/1(Sbp) -> Integrator/1
  Turbine exhaust system delay/1 -> Sum2/2
  MATLAB Function Acetogenesis/1(Xacidp) -> Integrator2/1
  Constant/1 -> Sum/2
  Constant18/1 -> MATLAB Function metano/5(Ksc)
  In1/1 -> MATLAB Function Acidogenesis/4(Ffeed), MATLAB Function metanogenesis/4(Ffeed), MATLAB Function Acetogenesis/4(Ffeed), MATLAB Function Hidrolisis/4(Ffeed)
  Add3/1 -> Product3/1, Product2/2
  [um] -> MATLAB Function Acetogenesis/5(um)
  Product3/1 -> Add4/1
  Constant15/1 -> MATLAB Function Acetogenesis/7(Ks)
  thermo couple/1 -> Scope8/1, Sum3/1
  Fuel system actuator/1 -> Delay combustor/1
  Add/1 -> Valve Positioner/1
  Add5/1 -> thermo couple/1
  Gain2/1 -> Add5/1
  Constant22/1 -> Product2/1
  [um] -> MATLAB Function metano/4(umc)
  Compresor/1 -> Add1/1
  Constant10/1 -> MATLAB Function Acidogenesis/13(Ksc)
  [um] -> MATLAB Function Acidogenesis/6(umc), MATLAB Function Acidogenesis/5(um)
  Constant9/1 -> MATLAB Function Acidogenesis/11(Ks)
  Constant1/1 -> Gain/1
  Constant13/1 -> MATLAB Function metanogenesis/8(Kdc)
  Constant26/1 -> Sum3/2, Add4/3
  Integrator1/1 -> Scope2/1, [Sv]
  [Xmeth] -> MATLAB Function metanogenesis/1(Xmeth)
  Add2/1 -> Gain3/1  "Torque mecánico"
  MATLAB Function/1(y) -> Delay combustor1/1
  Saturation/1 -> Vdc/1, Scope9/1
  [Sb] -> MATLAB Function Hidrolisis/2(Sb)
  Min/1 -> Product/1
  Constant3/1 -> [V], MATLAB Function Hidrolisis/3(V)
  MATLAB Function Acidogenesis/1(Svp) -> Integrator1/1
  Constant5/1 -> MATLAB Function Hidrolisis/1(Sbin)
  Constant20/1 -> Product1/2
  [Xmeth] -> MATLAB Function Acidogenesis/10(Xmeth)
  Sum3/1 -> Temp Control/1
  Gain1/1 -> Saturation/1
  Constant21/1 -> Add3/1
  Constant25/1 -> Sum2/1
  Product2/1 -> Add2/2
  [Xacid] -> MATLAB Function Acidogenesis/9(Xacid)
  Valve Positioner/1 -> Fuel system actuator/1
  Constant4/1 -> MATLAB Function Hidrolisis/6(K1)
  Constant11/1 -> MATLAB Function metanogenesis/2(b)
  Rotation Shield/1 -> Add5/2
  Add1/1 -> Product1/1
  [Sv] -> MATLAB Function Acidogenesis/2(Sv)
  [Xacid] -> MATLAB Function Acetogenesis/1(Xacid)
  Constant19/1 -> Add1/2
  Product1/1 -> Add2/1
  Transfer Fcn/1 -> Min/1
  Delay combustor1/1 -> Add/2
  [um] -> MATLAB Function metanogenesis/5(umc)
  MATLAB Function metanogenesis/1(Xmethp) -> Integrator3/1
  Constant14/1 -> MATLAB Function metanogenesis/6(Ksc)
  Product4/1 -> Add4/2
  Constant2/1 -> MATLAB Function Hidrolisis/8(Ks)
  Constant17/1 -> MATLAB Function metano/2(K4)
  [V] -> MATLAB Function metano/3(V)
  [Xmeth] -> MATLAB Function metano/1(Xmeth)
  [Xacid] -> MATLAB Function Hidrolisis/7(Xacid)
  Delay/1 -> Add3/2

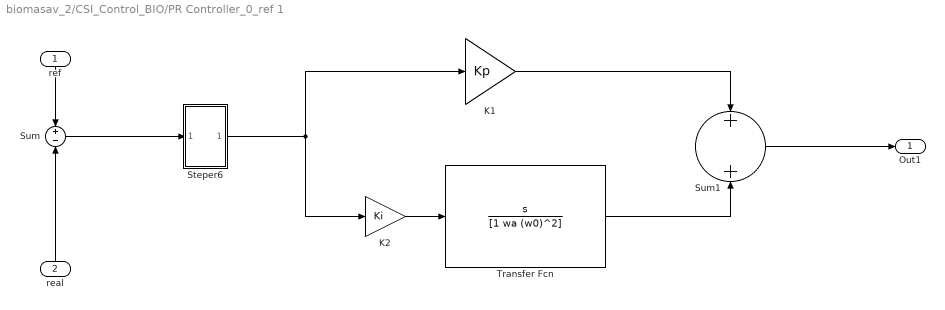
== system biomasav_2/CSI_Control_BIO/PR Controller_0_ref 1 ==
  ref : Inport
  real : Inport  Port=2
  K1 : Gain  Gain=Kp
  K2 : Gain  Gain=Ki
  Steper6 : Subsystem
  Sum : Sum  Inputs=+-
  Sum1 : Sum  Inputs=+|+
  Transfer Fcn : TransferFcn  Numerator=[1 0]  Denominator=[1 wa (w0)^2]
  Out1 : Outport
  wires:
  real/1 -> Sum/2
  ref/1 -> Sum/1
  Sum/1 -> Steper6/1(In1)
  K1/1 -> Sum1/1
  Transfer Fcn/1 -> Sum1/2
  K2/1 -> Transfer Fcn/1
  Steper6/1(Out1) -> K1/1, K2/1
  Sum1/1 -> Out1/1

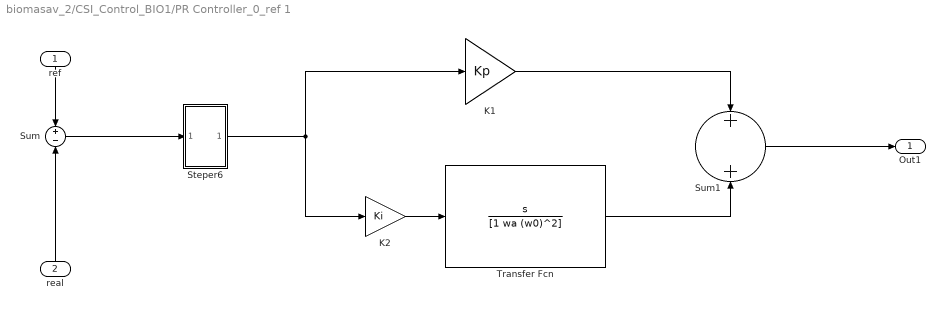
== system biomasav_2/CSI_Control_BIO1/PR Controller_0_ref 1 ==
  ref : Inport
  real : Inport  Port=2
  K1 : Gain  Gain=Kp
  K2 : Gain  Gain=Ki
  Steper6 : Subsystem
  Sum : Sum  Inputs=+-
  Sum1 : Sum  Inputs=+|+
  Transfer Fcn : TransferFcn  Numerator=[1 0]  Denominator=[1 wa (w0)^2]
  Out1 : Outport
  wires:
  real/1 -> Sum/2
  ref/1 -> Sum/1
  Sum/1 -> Steper6/1(In1)
  K1/1 -> Sum1/1
  Transfer Fcn/1 -> Sum1/2
  K2/1 -> Transfer Fcn/1
  Steper6/1(Out1) -> K1/1, K2/1
  Sum1/1 -> Out1/1

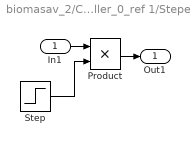
== system biomasav_2/CSI_Control_BIO/PR Controller_0_ref 1/Steper6 ==
  In1 : Inport
  Product : Product
  Step : Step  Time=st_time  SampleTime=0
  Out1 : Outport
  wires:
  Product/1 -> Out1/1
  In1/1 -> Product/1
  Step/1 -> Product/2

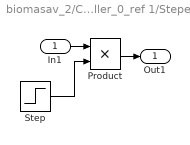
== system biomasav_2/CSI_Control_BIO1/PR Controller_0_ref 1/Steper6 ==
  In1 : Inport
  Product : Product
  Step : Step  Time=st_time  SampleTime=0
  Out1 : Outport
  wires:
  Product/1 -> Out1/1
  In1/1 -> Product/1
  Step/1 -> Product/2

== matlab function biomasav_2/CSI_Control_BIO/PQ_singlePhase ==
  data: va input; p output; vb input; ia input; ib input; q output
function [p, q] = fcn(va, vb, ia, ib)
% Esta funcion calcula la potencia activa y reactiva instantanea
% para el caso mnosofasico. En la revision de 2 papers he observado
% que una manera de extender la teoria de potencia al caso monofasico
% es asumiendo la tension o corriente de una fase como la componente
% alpha y hacer un desfase de 90 grados para obtener una version
% artificial de beta.

paux=va*ia+vb*ib;
if(paux > 20e4)
    paux = 20e4;
end
if(paux < -20e4)
    paux = -20e-4;
end

p = paux/2; % potencia activa instantanea

qaux = vb*ia-va*ib;

if(qaux>20e4)
    qaux=20e4;
end
if(qaux<-20e4)
    qaux=-20e4;
end

q = qaux/2; % potencia reactiva instantanea

== matlab function biomasav_2/CSI_Control_BIO1/PQ2Iab_PH1 ==
  data: Va input; Ia output; Vb input; p input; q input; Ib output
function [Ia, Ib] = fcn(Va, Vb, p, q)
%#codegen
% Ia=0;
% Ib=0;
% divide by zero protection
if(abs((Va^2+Vb^2))<=1000*eps(0))
    det = 1/eps(0);
else
    det = 1/(Va^2+Vb^2); % constante auxiliar
end
%det = 1/(Va^2+Vb^2);

Mat = det*[Va Vb; Vb -Va];

Iab = Mat*[2*p;2*q];

Iaaux = Iab(1);
Ibaux = Iab(2);

ilim=1e3;

if(Iaaux>ilim)
    Iaaux=ilim;
end
if(Iaaux<-ilim)
    Iaaux =-ilim;    
end

if(isnan(Iaaux))
    Iaaux=0;
end
%-----------------


if(Ibaux>ilim)
    Ibaux=ilim;
end
if(Ibaux<-ilim)
    Ibaux =-ilim;    
end

if(isnan(Ibaux))
    Ibaux=0;
end
%-----------------


Ia = Iaaux;
Ib = Ibaux;

== matlab function biomasav_2/CSI_Control_BIO1/PQ_singlePhase ==
  data: va input; p output; vb input; ia input; ib input; q output
function [p, q] = fcn(va, vb, ia, ib)
% Esta funcion calcula la potencia activa y reactiva instantanea
% para el caso mnosofasico. En la revision de 2 papers he observado
% que una manera de extender la teoria de potencia al caso monofasico
% es asumiendo la tension o corriente de una fase como la componente
% alpha y hacer un desfase de 90 grados para obtener una version
% artificial de beta.

paux=va*ia+vb*ib;
if(paux > 20e4)
    paux = 20e4;
end
if(paux < -20e4)
    paux = -20e-4;
end

p = paux/2; % potencia activa instantanea

qaux = vb*ia-va*ib;

if(qaux>20e4)
    qaux=20e4;
end
if(qaux<-20e4)
    qaux=-20e4;
end

q = qaux/2; % potencia reactiva instantanea

== matlab function biomasav_2/MATLAB Function3 ==
  data: w input; y output; torque input; potencia input
function y = fcn(w,torque,potencia)
%#codegen

y = w*torque*1000/potencia;

== matlab function biomasav_2/MATLAB Function SOC  ==
  data: u input; y output
function y = fcn(u)

y = -0.03536*u+100;

== matlab function biomasav_2/CSI_Control_BIO/PQ2Iab_PH1 ==
  data: Va input; Ia output; Vb input; p input; q input; Ib output
function [Ia, Ib] = fcn(Va, Vb, p, q)
%#codegen
% Ia=0;
% Ib=0;
% divide by zero protection
if(abs((Va^2+Vb^2))<=1000*eps(0))
    det = 1/eps(0);
else
    det = 1/(Va^2+Vb^2); % constante auxiliar
end
%det = 1/(Va^2+Vb^2);

Mat = det*[Va Vb; Vb -Va];

Iab = Mat*[2*p;2*q];

Iaaux = Iab(1);
Ibaux = Iab(2);

ilim=1e3;

if(Iaaux>ilim)
    Iaaux=ilim;
end
if(Iaaux<-ilim)
    Iaaux =-ilim;    
end

if(isnan(Iaaux))
    Iaaux=0;
end
%-----------------


if(Ibaux>ilim)
    Ibaux=ilim;
end
if(Ibaux<-ilim)
    Ibaux =-ilim;    
end

if(isnan(Ibaux))
    Ibaux=0;
end
%-----------------


Ia = Iaaux;
Ib = Ibaux;

== matlab function biomasav_2/MATLAB Function5 ==
  data: p input; y output; q input
function y = fcn(p,q)

y = sqrt(p^2+q^2);

== matlab function biomasav_2/MATLAB Function6 ==
  data: p input; y output; q input
function y = fcn(p,q)

y = sqrt(p^2+q^2);

== matlab function biomasav_2/MeasureNode_I1/MATLAB Function ==
  data: u1 input; y output; u2 input; y2 output
function [y,y2] = fcn(u1,u2)

if (u1>=1 && u1<=1.3) || (u1>=2.5 && u1<=2.8)%u1>=1000
    y=u2+u2*0.35;
    y2=u2*0.35;
else
    y = u2;
    y2=0;
end

== matlab function biomasav_2/generador biomasa/MATLAB Function ==
  data: u1 input; y output; u2 input
function y = fcn(u1,u2)

y = u2*(1-u1);

== matlab function biomasav_2/generador biomasa/MATLAB Function Acetogenesis ==
  data: Xacid input; b input; V input; Ffeed input; um input; Kd input; Ks input; Xacidp output; Sb input
function Xacidp = fcn(Xacid,b,V,Ffeed,um,Kd,Ks,Sb)

% Xacidp=(um/(1+Ks/Sb)-Kd-Ffeed/(b*V))*Xacid;
Xacidp=(um/(Ks/(1+Sb))-Kd-Ffeed/(b*V))*Xacid;

== matlab function biomasav_2/generador biomasa/MATLAB Function Acidogenesis ==
  data: Svin input; Sv input; V input; Ffeed input; um input; umc input; K2 input; K3 input; Xacid input; Xmeth input; Ks input; Svp output; Sb input; Ksc input
function Svp = fcn(Svin,Sv,V,Ffeed,um,umc,K2,K3,Xacid,Xmeth,Ks,Sb,Ksc)

% Svp=(Svin-Sv)*(Ffeed/V)+um*K2*Xacid/(1+Ks/Sb)-umc*K3*Xmeth/(1+Ksc/Sv);
Svp=(Svin-Sv)*(Ffeed/V)+um*K2*Xacid/(Ks/(1+Sb))-umc*K3*Xmeth/(Ksc/(1+Sv));

== matlab function biomasav_2/generador biomasa/MATLAB Function Hidrolisis ==
  data: Sbin input; Sbp output; Sb input; V input; Ffeed input; um input; K1 input; Xacid input; Ks input
function Sbp = fcn(Sbin,Sb,V,Ffeed,um,K1,Xacid,Ks)

% Sbp=(Sbin-Sb)*(Ffeed/V)+um*K1*Xacid/(1+Ks/Sb);
Sbp=(Sbin-Sb)*(Ffeed/V)+um*K1*Xacid/(Ks/(1+Sb));

== matlab function biomasav_2/generador biomasa/MATLAB Function metano ==
  data: Xmeth input; K4 input; V input; umc input; Ksc input; Sv input; Fmeth output
function Fmeth = fcn(Xmeth,K4,V,umc,Ksc,Sv)


% Fmeth=V*umc*K4*Xmeth/(Ksc/Sv+1);
Fmeth=V*umc*K4*Xmeth/(Ksc/(Sv+1));

== matlab function biomasav_2/generador biomasa/MATLAB Function metanogenesis ==
  data: Xmeth input; b input; V input; Ffeed input; umc input; Ksc input; Sv input; Xmethp output; Kdc input
function Xmethp = fcn(Xmeth,b,V,Ffeed,umc,Ksc,Sv,Kdc)

% Xmethp=(umc/(Ksc/Sv+1)-Kdc-Ffeed/(b*V))*Xmeth;
Xmethp=(umc/(Ksc/(Sv+1))-Kdc-Ffeed/(b*V))*Xmeth;
